simulink model "mod5"  (R2020a)
settings: Solver=FixedStepDiscrete  StartTime=0.0  StopTime=10  MaxStep=0.2  RelTol=1e-3
settings Model: EnablePacing=on  PacingRate=0.400000  Creator=I3  LastModifiedBy=I3

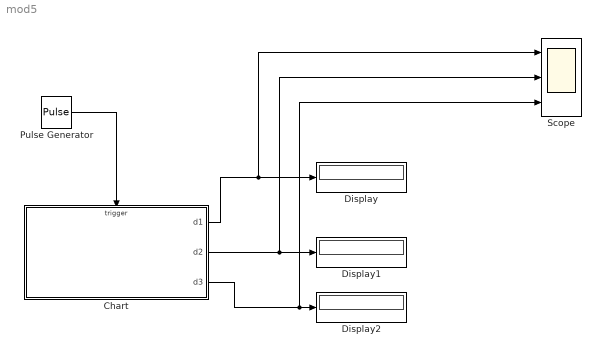
== system mod5 ==
  Chart : Stateflow chart  TreatAsAtomicUnit=on
  Display : Display
  Display1 : Display
  Display2 : Display
  Pulse Generator : DiscretePulseGenerator  PulseType=Time based  Period=10  PulseWidth=5
  Scope : Scope  NumInputPorts=3
  wires:
  Pulse Generator/1 -> Chart/Trigger
  Chart/1(d1) -> Scope/1, Display/1
  Chart/3(d3) -> Scope/3, Display2/1
  Chart/2(d2) -> Scope/2, Display1/1

== stateflow chart mod5/Chart ==
  state digit1 [parallel]
    settings: executionOrder=1
    state four
      en:
      d1=4;
    state three
      en:
      d1=3;
    state zero
      en:
      d1=0;
    state one
      en:
      d1=1;
    state two
      en:
      d1=2;
    (default) -> digit1.zero
    digit1.one -> digit1.two : inc1
    digit1.zero -> digit1.one : inc1
    digit1.two -> digit1.three : inc1
    digit1.three -> digit1.four : inc1
    digit1.four -> digit1.zero : inc1/{inc2}
  state digit3 [parallel]
    settings: executionOrder=3
    state four
      en:
      d1=4;
    state three
      en:
      d3=3;
    state zero
      en:
      d3=0;
    state one
      en:
      d3=1;
    state two
      en:
      d3=2;
    (default) -> digit3.zero
    digit3.one -> digit3.two : inc3
    digit3.zero -> digit3.one : inc3
    digit3.two -> digit3.three : inc3
    digit3.three -> digit3.four : inc3
    digit3.four -> digit3.zero : inc3
  state digit2 [parallel]
    settings: executionOrder=2
    state four
      en:
      d2=4;
    state three
      en:
      d2=3;
    state zero
      en:
      d2=0;
    state one
      en:
      d2=1;
    state two
      en:
      d2=2;
    (default) -> digit2.zero
    digit2.one -> digit2.two : inc2
    digit2.zero -> digit2.one : inc2
    digit2.two -> digit2.three : inc2
    digit2.three -> digit2.four : inc2
    digit2.four -> digit2.zero : inc2/{inc3}
  data: d1 output; d2 output; d3 output
  events: inc2 local FUNCTION_CALL_EVENT; inc3 local FUNCTION_CALL_EVENT; inc1 input RISING_EDGE_EVENT
